simulink model "model1"  (R2014a)
settings: Solver=ode4  StartTime=0.0  StopTime=100.0  FixedStep=0.01  RelTol=1e-3
settings Model: Creator=Cula  LastModifiedBy=Cula

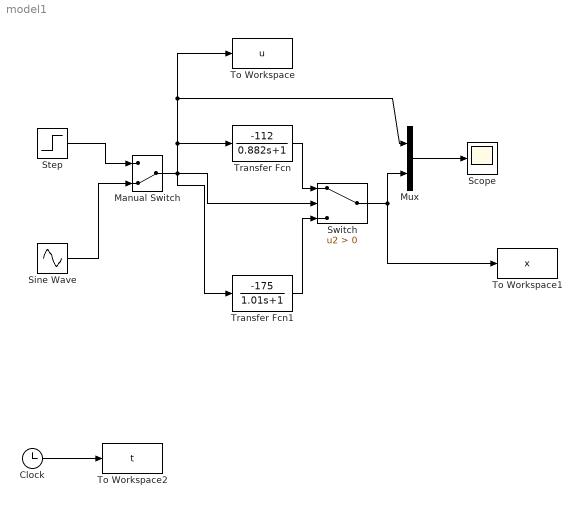
== system model1 ==
  Clock : Clock
  Manual Switch : ManualSwitch  CurrentSetting=0
  Mux : Mux  Inputs=2
  Scope : Scope
  Sine Wave : Sin  Amplitude=10  Frequency=0.1  SampleTime=0
  Step : Step  SampleTime=0
  Switch : Switch  Criteria=u2 > Threshold
  To Workspace : ToWorkspace  VariableName=u  SaveFormat=Timeseries  SampleTime=-1
  To Workspace1 : ToWorkspace  VariableName=x  SaveFormat=Timeseries  SampleTime=-1
  To Workspace2 : ToWorkspace  VariableName=t  SaveFormat=Timeseries  SampleTime=-1
  Transfer Fcn : TransferFcn  Numerator=[-112]  Denominator=[0.882 1]
  Transfer Fcn1 : TransferFcn  Numerator=[-175]  Denominator=[1.01 1]
  wires:
  Step/1 -> Manual Switch/1
  Sine Wave/1 -> Manual Switch/2
  Manual Switch/1 -> Transfer Fcn1/1, Switch/2, Transfer Fcn/1, To Workspace/1, Mux/1
  Mux/1 -> Scope/1
  Clock/1 -> To Workspace2/1
  Switch/1 -> To Workspace1/1, Mux/2
  Transfer Fcn/1 -> Switch/1
  Transfer Fcn1/1 -> Switch/3
